simulink model "parameters_identification_21a"  (R2021a)
settings: Solver=VariableStepAuto  StartTime=0.0  StopTime=10.0  RelTol=1e-3
settings Model: Creator=Guilherme  LastModifiedBy=carol
settings DebuggingCC: UnconnectedInputMsg=none  UnconnectedOutputMsg=none  UnconnectedLineMsg=none
settings ModelReferenceCC: EnableRefExpFcnMdlSchedulingChecks=off
settings RTWCC: Description=Generic Real-Time Target  GPUComputeCapability=5.0  DLArmComputeVersion=20.02.1

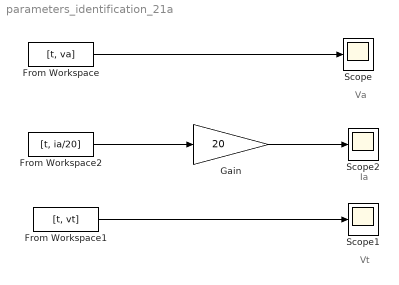
== system parameters_identification_21a ==
  note: Ia
  note: Va
  note: Vt
  From Workspace : FromWorkspace  VariableName=[t, va]
  From Workspace1 : FromWorkspace  VariableName=[t, vt]
  From Workspace2 : FromWorkspace  VariableName=[t, ia/20]
  Gain : Gain  Gain=20
  Scope : Scope
  Scope1 : Scope
  Scope2 : Scope
  wires:
  From Workspace/1 -> Scope/1
  From Workspace1/1 -> Scope1/1
  From Workspace2/1 -> Gain/1
  Gain/1 -> Scope2/1
